simulink library "Transmission_Lib_org"  (Simulink 10.0)
settings: Solver=ode45  StartTime=0.0  StopTime=10.0  RelTol=1e-3  EnableMultiTasking=on
undefined symbols (not defined in the file): DCT_Param
libraries: fl_lib x45, nesl_utility x25, sdl_lib x18, Animation_Lib x2, $bdroot x1
(part 2 of 2)

== system Transmission_Lib_org/Detailed/Gears/Sensing5 ==
  PS-Simulink Converter : nesl_utility/PS-Simulink Converter  PhysicalDomain=network_engine_domain  SubClassName=ps_output  LeftPortType=input  RightPortType=output  PseudoPeriodic=off  Frequencies=[]  Unit=1  AffineConversion=off
  S : PMIOPort  Side=Left
  tag scope: DCT_Cl2_Disp=global
  wires:
  PS-Simulink Converter/1 -> [DCT_Cl2_Disp]
  connections:
  S/RConn1 -- PS-Simulink Converter/LConn1

== system Transmission_Lib_org/Detailed/Gears/Sensing6 ==
  PS-Simulink Converter : nesl_utility/PS-Simulink Converter  PhysicalDomain=network_engine_domain  SubClassName=ps_output  LeftPortType=input  RightPortType=output  PseudoPeriodic=off  Frequencies=[]  Unit=1  AffineConversion=off
  S : PMIOPort  Side=Left
  tag scope: DCT_Cl3_Disp=global
  wires:
  PS-Simulink Converter/1 -> [DCT_Cl3_Disp]
  connections:
  S/RConn1 -- PS-Simulink Converter/LConn1

== system Transmission_Lib_org/Detailed/Gears/Sensing7 ==
  PS-Simulink Converter : nesl_utility/PS-Simulink Converter  PhysicalDomain=network_engine_domain  SubClassName=ps_output  LeftPortType=input  RightPortType=output  PseudoPeriodic=off  Frequencies=[]  Unit=1  AffineConversion=off
  S : PMIOPort  Side=Left
  tag scope: DCT_Cl4_Disp=global
  wires:
  PS-Simulink Converter/1 -> [DCT_Cl4_Disp]
  connections:
  S/RConn1 -- PS-Simulink Converter/LConn1

== system Transmission_Lib_org/Detailed/Gears/Sensing8 ==
  PS-Simulink Converter : nesl_utility/PS-Simulink Converter  PhysicalDomain=network_engine_domain  SubClassName=ps_output  LeftPortType=input  RightPortType=output  PseudoPeriodic=off  Frequencies=[]  Unit=1  AffineConversion=off
  S : PMIOPort  Side=Left
  tag scope: DCT_Cl5_Disp=global
  wires:
  PS-Simulink Converter/1 -> [DCT_Cl5_Disp]
  connections:
  S/RConn1 -- PS-Simulink Converter/LConn1

== system Transmission_Lib_org/Detailed/Gears/Sensing9 ==
  PS-Simulink Converter : nesl_utility/PS-Simulink Converter  PhysicalDomain=network_engine_domain  SubClassName=ps_output  LeftPortType=input  RightPortType=output  PseudoPeriodic=off  Frequencies=[]  Unit=1  AffineConversion=off
  S : PMIOPort  Side=Left
  tag scope: DCT_Cl6_Disp=global
  wires:
  PS-Simulink Converter/1 -> [DCT_Cl6_Disp]
  connections:
  S/RConn1 -- PS-Simulink Converter/LConn1

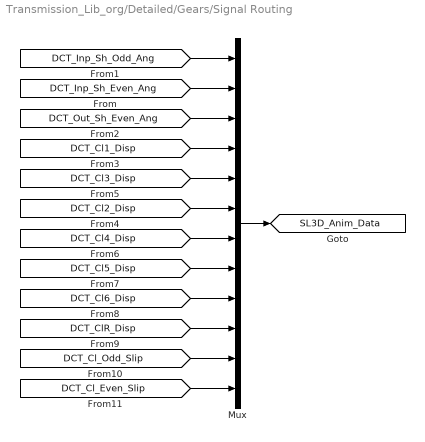
== system Transmission_Lib_org/Detailed/Gears/Signal Routing ==
  Mux : Mux  Inputs=12
  tag scope: SL3D_Anim_Data=global
  wires:
  [DCT_Cl_Even_Slip] -> Mux/12
  [DCT_Cl_Odd_Slip] -> Mux/11
  [DCT_ClR_Disp] -> Mux/10
  [DCT_Cl6_Disp] -> Mux/9
  [DCT_Cl5_Disp] -> Mux/8
  [DCT_Cl4_Disp] -> Mux/7
  [DCT_Cl2_Disp] -> Mux/6
  [DCT_Cl3_Disp] -> Mux/5
  [DCT_Cl1_Disp] -> Mux/4
  [DCT_Out_Sh_Even_Ang] -> Mux/3
  [DCT_Inp_Sh_Odd_Ang] -> Mux/1
  [DCT_Inp_Sh_Even_Ang] -> Mux/2
  Mux/1 -> [SL3D_Anim_Data]

== system Transmission_Lib_org/Abstracted/Gears/Ratio Selection/Lag Filter with IC ==
  In : Inport
  Gain : Gain  Gain=1/b
  Integrator : Integrator  InitialCondition=x_initial*b
  Sum : Sum  Inputs=|+-  SaturateOnIntegerOverflow=on  InputSameDT=on  OutDataTypeStr=Inherit: Same as first input
  Out : Outport
  wires:
  Gain/1 -> Out/1, Sum/2
  Integrator/1 -> Gain/1
  In/1 -> Sum/1
  Sum/1 -> Integrator/1

== system Transmission_Lib_org/Detailed/Clutches/Slip sensor 1/Sensing4 ==
  S : Inport
  tag scope: DCT_Cl_Odd_Slip=global
  wires:
  S/1 -> [DCT_Cl_Odd_Slip]

== system Transmission_Lib_org/Detailed/Clutches/Slip sensor 2/Sensing4 ==
  S : Inport
  tag scope: DCT_Cl_Even_Slip=global
  wires:
  S/1 -> [DCT_Cl_Even_Slip]
